simulink model "SailingYachtModelUpdated2"  (R2023b)
settings: Solver=ode3  StartTime=0.0  StopTime=200  FixedStep=0.05  RelTol=1e-3  EnableMultiTasking=on
undefined symbols (not defined in the file or in its folder): par
libraries: simulink_extras x12, vrlib x3
settings Model: Creator=Administrator  LastModifiedBy=henri
settings SolverCC: AlgebraicLoopSolver=TrustRegion
settings DataIOCC: LimitDataPoints=on  SaveFormat=Array  SignalLoggingSaveFormat=ModelDataLogs  ReturnWorkspaceOutputs=off
settings OptimizationCC: ExpressionDepthLimit=2147483647  InitFltsAndDblsToZero=on  LifeSpan=inf
settings DebuggingCC: SaveWithParameterizedLinksMsg=none  UnderspecifiedInitializationDetection=Classic  MergeDetectMultiDrivingBlocksExec=none  SignalResolutionControl=TryResolveAllWithWarning  SolverPrmCheckMsg=warning  MultiTaskDSMMsg=warning  MultiTaskCondExecSysMsg=none  FcnCallInpInsideContextMsg=warning  UnconnectedInputMsg=warning  UnconnectedOutputMsg=warning  UnconnectedLineMsg=warning  StateNameClashWarn=warning  SFUnexpectedBacktrackingDiag=warning  SFNoUnconditionalDefaultTransitionDiag=warning  SFExecutionAtInitializationDiag=none  ArithmeticOperatorsInVariantConditions=warning
settings HardwareCC: ProdBitPerPointer=32  ProdBitPerSizeT=32  ProdBitPerPtrDiffT=32  ProdLargestAtomicFloat=None  ProdIntDivRoundTo=Undefined  ProdEndianess=Unspecified  ProdWordSize=32  ProdHWDeviceType=32-bit Generic
settings ModelReferenceCC: PropagateSignalLabelsOutOfModel=off
settings SFSimCC: SimUseLocalCustomCode=off  CustomCodeUndefinedFunction=UseInterfaceOnly
settings RTWCC: RTWUseLocalCustomCode=off
settings CodeAppCC: StateflowObjectComments=on
settings GRTTargetCC: TargetFcnLib=ansi_tfl_tmw.mat  TargetLangStandard=C89/C90 (ANSI)  CombineOutputUpdateFcns=off  GRTInterface=on
settings ConfigComp: CovMetricSettings=dw  CovSaveCumulativeToWorkspaceVar=on  CovSaveSingleToWorkspaceVar=on  CovExternalEMLEnable=off

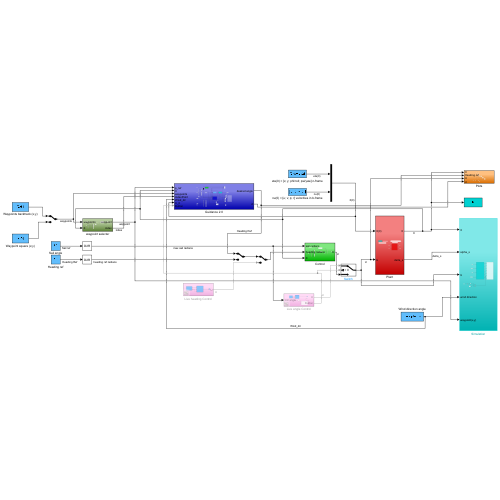
[thumbnail: Simulink's stored preview of the top-level diagram]
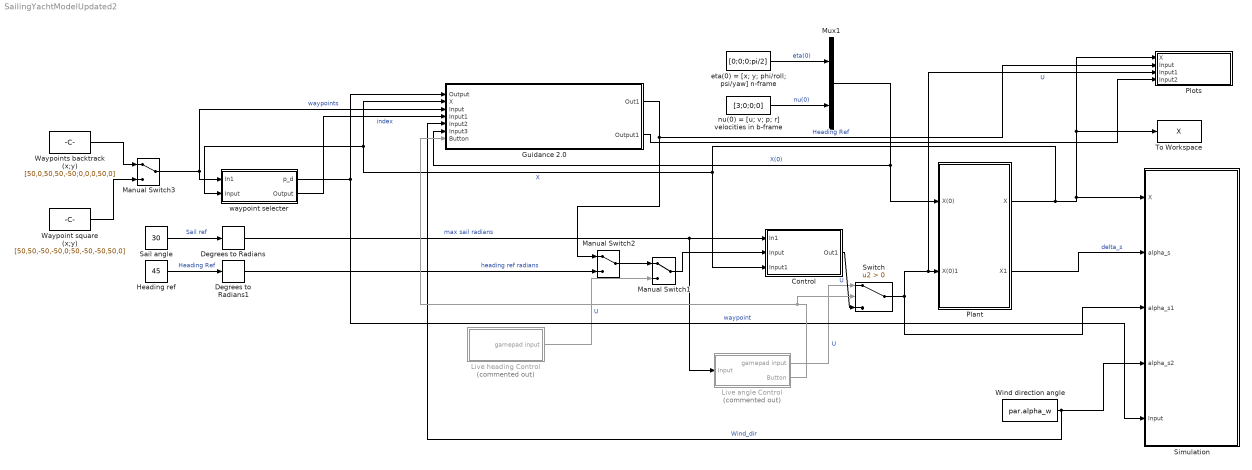
== system SailingYachtModelUpdated2 ==
  Control : Subsystem
  Degrees to Radians : simulink_extras/Transformations/Degrees to Radians
  Degrees to Radians1 : simulink_extras/Transformations/Degrees to Radians
  Guidance 2.0 : Subsystem
  Heading ref : Constant  Value=45
  Live angle Control : Subsystem  Commented=on
  Live heading Control : Subsystem  Commented=on
  Manual Switch1 : ManualSwitch
  Manual Switch2 : ManualSwitch
  Manual Switch3 : ManualSwitch
  Mux1 : Mux  Inputs=2
  Plant : Subsystem
  Plots : Subsystem
  Sail angle : Constant  Value=30
  Simulation : Subsystem
  Switch : Switch  Criteria=u2 > Threshold  SaturateOnIntegerOverflow=off  InputSameDT=off
  To Workspace : ToWorkspace  VariableName=X  SaveFormat=Structure With Time  SampleTime=-1
  Waypoint square (x;y) : Constant  Value=[50,50,-50,-50,0;50,-50,-50,50,0]  VectorParams1D=off
  Waypoints backtrack (x;y) : Constant  Value=[50,0,50,50,-50;0,0,0,50,0]  VectorParams1D=off
  Wind direction angle : Constant  Value=par.alpha_w
  eta(0) = [x; y; phi/roll; psi/yaw] n-frame : Constant  Value=[0;0;0;pi/2]
  nu(0) = [u; v; p; r] velocities in b-frame : Constant  Value=[3;0;0;0]
  waypoint selecter : Subsystem
  wires:
  Mux1/1 -> Plant/1(X(0)), Guidance 2.0/6(Input3)  "X(0)"
  Switch/1 -> Plots/3(Input1), Plant/2(X(0)1), Simulation/3(alpha_s1)  "U"
  Plant/1(X) -> Guidance 2.0/2(X), waypoint selecter/2(Input), Control/3(Input1), Plots/1(X), To Workspace/1, Simulation/1(X)  "X"
  Heading ref/1 -> Degrees to Radians1/1  "Heading Ref"
  Plant/2(X1) -> Simulation/2(alpha_s)  "delta_s"
  Wind direction angle/1 -> Guidance 2.0/5(Input2), Simulation/4(alpha_s2)  "Wind_dir"
  eta(0) = [x; y; phi/roll; psi/yaw] n-frame/1 -> Mux1/1  "eta(0)"
  nu(0) = [u; v; p; r] velocities in b-frame/1 -> Mux1/2  "nu(0)"
  Degrees to Radians/1 -> Live angle Control/1(Input), Control/1(In1)  "max sail radians"
  Sail angle/1 -> Degrees to Radians/1  "Sail ref"
  Degrees to Radians1/1 -> Manual Switch2/2  "heading ref radians"
  Live angle Control/1(gamepad input) -> Switch/1  "U"
  Control/1(Out1) -> Switch/3  "U"
  Live heading Control/1(gamepad input) -> Manual Switch1/2  "U"
  Manual Switch1/1 -> Control/2(Input)
  Manual Switch2/1 -> Manual Switch1/1
  waypoint selecter/1(p_d) -> Simulation/5(Input), Guidance 2.0/1(Output)  "waypoint"
  waypoint selecter/2(Output) -> Guidance 2.0/4(Input1)  "index"
  Guidance 2.0/1(Out1) -> Manual Switch2/1, Plots/2(Input)  "Heading Ref"
  Manual Switch3/1 -> waypoint selecter/1(In1), Guidance 2.0/3(Input)  "waypoints"
  Waypoint square (x;y)/1 -> Manual Switch3/2
  Waypoints backtrack (x;y)/1 -> Manual Switch3/1
  Guidance 2.0/2(Output1) -> Plots/4(Input2)
  Live angle Control/2(Button) -> Switch/2, Guidance 2.0/7(Button)

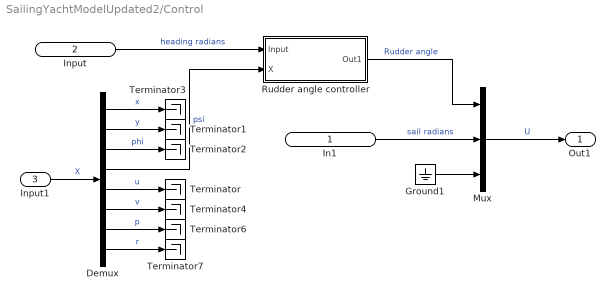
== system SailingYachtModelUpdated2/Control ==
  In1 : Inport
  Input : Inport  Port=2
  Input1 : Inport  Port=3
  Demux : Demux  Outputs=8
  Ground1 : Ground
  Mux : Mux  Inputs=3
  Rudder angle controller : Subsystem
  Terminator{,1..4,6..7} (7 alike) : Terminator
  Out1 : Outport
  wires:
  In1/1 -> Mux/2  "sail radians"
  Rudder angle controller/1(Out1) -> Mux/1  "Rudder angle"
  Mux/1 -> Out1/1  "U"
  Input/1 -> Rudder angle controller/1(Input)  "heading radians"
  Input1/1 -> Demux/1  "X"
  Demux/1 -> Terminator3/1  "x"
  Demux/2 -> Terminator1/1  "y"
  Demux/3 -> Terminator2/1  "phi"
  Demux/4 -> Rudder angle controller/2(X)  "psi"
  Demux/5 -> Terminator/1  "u"
  Demux/6 -> Terminator4/1  "v"
  Demux/7 -> Terminator6/1  "p"
  Demux/8 -> Terminator7/1  "r"
  Ground1/1 -> Mux/3

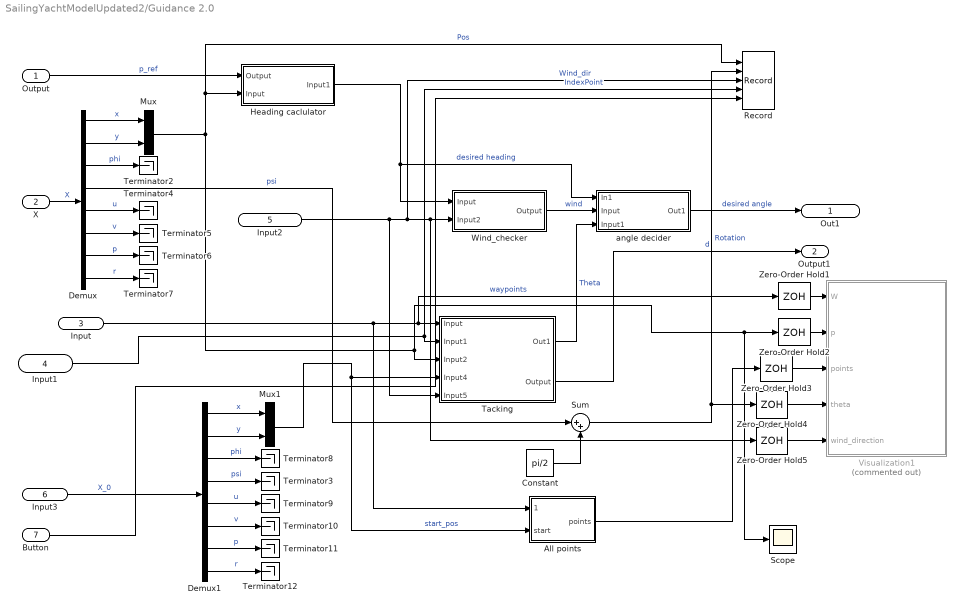
== system SailingYachtModelUpdated2/Guidance 2.0 ==
  Output : Inport
  X : Inport  Port=2
  Input : Inport  Port=3
  Input1 : Inport  Port=4
  Input2 : Inport  Port=5
  Input3 : Inport  Port=6
  Button : Inport  Port=7
  All points : MATLAB Function  TreatAsAtomicUnit=on
  Constant : Constant  Value=pi/2
  Demux : Demux  Outputs=8
  Demux1 : Demux  Outputs=8
  Heading caclulator : Subsystem
  Mux : Mux  Inputs=2
  Mux1 : Mux  Inputs=2
  Record : Record  Filename=C:\Users\henri\OneDrive - Syddansk Universitet\8. Semester\GNC\Assignment_finalV3\AutoRouteFrontBack.xlsx  RecordToFile=on  FileSettingsInternal="{\"entries\":[{\"content\":{\"excelSettings\":{\"content\":{},\"type\":\"Streamout.ExcelSettings\"}},\"type\":\"Streamout.FileSettingStorage\",\"uuid\":\"\"}],\"packageUris\":[\"http:\\/\\/schema.mathworks.com\\/mf0\\/streamout_blocks\\/R2020a\"],\"version\":\"1.0\"}"  SignalsInternal="{\"entries\":[{\"content\":{\"signals\":[{\"content\":{\"blockPath\":[],\"dimensions\":[2],\"domain\":\"\",\"hasChildren\":true,\"lineColor\":\"#ff13a6\",\"port\":1,\"sid\":[\"\"],\"signalID\":899,\"signalName\":\"Pos\"},\"type\":\"RecordBlkView.Signal\",\"uuid\":\"\"},{\"content\":{\"blockPath\":[],\"channel\":[1],\"dimensions\":[2],\"domain\":\"\",\"lineColor\":\"#22b573\",\"parentID\":899,\"plots\":[1],\"port\":1,\"sid\":[\"\"],\"signalID\":900,\"signalName\":\"Pos\"},\"type\":\"RecordBlkView.Signal\",\"uuid\":\"\"},{\"content\":{\"blockPath\":[],\"dimensions\":[1],\"domain\":\"\",\"lineColor\":\"#139fff\",\"plots\":[1],\"port\":2,\"sid\":[\"\"],\"signalID\":904,\"signalName\":\"Rotation\"},\"type\":\"RecordBlkView.Signal\",\"uuid\":\"\"},{\"content\":{\"blockPath\":[],\"dimensions\":[1],\"domain\":\"\",\"lineColor\":\"#b746ff\",\"plots\":[1],\"port\":4,\"sid\":[\"\"],\"signalID\":908,\"signalName\":\"IndexPoint\"},\"type\":\"RecordBlkView.Signal\",\"uuid\":\"\"},{\"content\":{\"blockPath\":[],\"dimensions\":[1],\"domain\":\"\",\"lineColor\":\"#ff6929\",\"plots\":[1],\"port\":3,\"sid\":[\"\"],\"signalID\":912,\"signalName\":\"Wind_dir\"},\"type\":\"RecordBlkView.Signal\",\"uuid\":\"\"},{\"content\":{\"blockPath\":[],\"dimensions\":[1],\"domain\":\"\",\"lineColor\":\"#ff6929\",\"plots\":[1],\"port\":5,\"sid\":[\"\"],\"signalID\":916,\"signalName\":\"Button\"},\"type\":\"RecordBlkView.Signal\",\"uuid\":\"\"},{\"content\":{\"blockPath\":[],\"channel\":[2],\"dimensions\":[2],\"domain\":\"\",\"lineColor\":\"#7e2f8e\",\"parentID\":899,\"plots\":[1],\"port\":1,\"sid\":[\"\"],\"signalID\":921,\"signalName\":\"Pos\"},\"type\":\"RecordBlkView.Signal\",\"uuid\":\"\"}]},\"type\":\"RecordBlkView.InputSignals\",\"uuid\":\"\"}],\"packageUris\":[\"http:\\/\\/schema.mathworks.com\\/mf0\\/streamout_blocks\\/R2020a\"],\"version\":\"1.0\"}"  VisualizationBindings="{\"sparklinesplugin\":{\"info\":[{\"bindingParametersList\":[],\"subplotID\":1}]}}"
  Scope : Scope
  Sum : Sum  Inputs=|++
  Tacking : Subsystem
  Terminator{2..12} (11 alike) : Terminator
  Visualization1 : MATLAB Function  Commented=on  TreatAsAtomicUnit=on
  Wind_checker : Subsystem
  Zero-Order Hold{1..5} (5 alike) : ZeroOrderHold  SampleTime=0.1
  angle decider : Subsystem
  Out1 : Outport
  Output1 : Outport  Port=2
  wires:
  Output/1 -> Heading caclulator/1(Output)  "p_ref"
  Demux/8 -> Terminator7/1  "r"
  Demux/7 -> Terminator6/1  "p"
  Demux/4 -> Sum/1  "psi"
  Demux/3 -> Terminator2/1  "phi"
  Demux/5 -> Terminator4/1  "u"
  X/1 -> Demux/1  "X"
  Demux/2 -> Mux/2  "y"
  Demux/1 -> Mux/1  "x"
  Demux/6 -> Terminator5/1  "v"
  Mux/1 -> Record/1, Heading caclulator/2(Input), Scope/1, Zero-Order Hold2/1, Tacking/3(Input2)  "Pos"
  Input/1 -> All points/1(waypoints), Zero-Order Hold1/1, Tacking/1(Input)  "waypoints"
  Input1/1 -> Record/4, Tacking/2(Input1)  "IndexPoint"
  Heading caclulator/1(Input1) -> angle decider/1(In1), Wind_checker/1(Input)  "desired heading"
  Input2/1 -> Tacking/5(Input5), Record/3, Zero-Order Hold5/1, Wind_checker/2(Input2)  "Wind_dir"
  angle decider/1(Out1) -> Out1/1  "desired angle"
  Wind_checker/1(Output) -> angle decider/2(Input)  "wind"
  Tacking/1(Out1) -> angle decider/3(Input1)  "Theta"
  Input3/1 -> Demux1/1  "X_0"
  Demux1/5 -> Terminator9/1  "u"
  Demux1/3 -> Terminator8/1  "phi"
  Demux1/8 -> Terminator12/1  "r"
  Demux1/7 -> Terminator11/1  "p"
  Demux1/6 -> Terminator10/1  "v"
  Demux1/4 -> Terminator3/1  "psi"
  Demux1/1 -> Mux1/1  "x"
  Demux1/2 -> Mux1/2  "y"
  Mux1/1 -> All points/2(start), Tacking/4(Input4)  "start_pos"
  Constant/1 -> Sum/2
  All points/1(points) -> Zero-Order Hold3/1
  Zero-Order Hold1/1 -> Visualization1/1(W)
  Zero-Order Hold2/1 -> Visualization1/2(p)
  Zero-Order Hold3/1 -> Visualization1/3(points)
  Zero-Order Hold4/1 -> Visualization1/4(theta)
  Zero-Order Hold5/1 -> Visualization1/5(wind_direction)
  Sum/1 -> Zero-Order Hold4/1, Record/2  "Rotation"
  Tacking/2(Output) -> Output1/1  "d"
  Button/1 -> Record/5

== system SailingYachtModelUpdated2/Live angle Control ==
  Input : Inport
  Formatting : Subsystem
  Gamepad : vrlib/Joystick Input  joyid=1  adjustports=on  forcefeed=off
  MATLAB Function : MATLAB Function  TreatAsAtomicUnit=on
  Selector : Selector  InputPortWidth=10  IndexOptions=Index vector (dialog)  Indices=[5]  OutputSizes=1
  gamepad input : Outport
  Button : Outport  Port=2
  wires:
  Gamepad/2 -> Formatting/2(Buttons), Selector/1
  Gamepad/1 -> Formatting/1(Axes)
  Formatting/1(gamepad input) -> gamepad input/1  "U"
  Input/1 -> Formatting/4(Input)  "sail angle"
  ? -> Formatting/3(Point of View)
  Selector/1 -> MATLAB Function/1(input)
  MATLAB Function/1(output) -> Button/1

== system SailingYachtModelUpdated2/Live heading Control ==
  Formatting : Subsystem
  Gamepad : vrlib/Joystick Input  joyid=1  adjustports=on  forcefeed=off
  gamepad input : Outport
  wires:
  Gamepad/2 -> Formatting/2(Buttons)
  Gamepad/1 -> Formatting/1(Axes)
  Formatting/1(gamepad input) -> gamepad input/1  "U"
  ? -> Formatting/3(Point of View)

== system SailingYachtModelUpdated2/Plant ==
  note: Jerome Jouffroy, Jiaxi He and Lin Xiao,
      | University of Southern Denmark, 2014.
  note: (program tested in Matlab r2013a, Simulink 8.1, Simulink 3D Animation 7.0)
  note: Simulation of a 4DOF sailing yacht model
  note: (includes wind speed and direction)
  note: (to look at/change the parameters of the sailing yacht
      | model, right-click on this block, then select
      | "Properties.../Callbacks/InitFcn")
  X(0) : Inport
  X(0)1 : Inport  Port=2
  4DOF nonlinear sailing yacht model : Subsystem
  SubSystem2 : Subsystem  InitFcn=|
      | global par
      | par.m = 25900;                         % (kg),mass of the vehicle
      | par.Ixx = 133690;          
      | par.Izz = 24760;      
      | par.Ixz = 2180;                        % moment of inertia
      | par.a11 = 970;   
      | par.a22 = 17430; 
      | par.a44 = 106500;
      | par.a66 = 101650;
      | par.a24 = -13160;
      | par.a26 = -6190; 
      | par.a46 = 4730;                        % (kg),added mass coef.
      | 
      | par.vt = 10;                           % the norm of wind velocity
      | par.alpha_w = pi;                      % the direction of wind (coming from the north, ie going south)
      | 
      | par.rho_a = 1.2;                       % (kg/m^3), air density
      | par.As = 170;                          % (m^2), sail area
      | par.h0 = 0.0005;                       % (m), roughness height
      | par.h1 = 11.58;                        % (m), reference height
      | par.z_s = -11.58;                      % (m), (x,y,z) is the CoE
      | par.xs = 0;
      | par.ys = 0;
      | par.zs = -11.58;                       % (m), (x,y,z) is the CoE
      | par.Xce = 0.6;                         % (m), distance along the mast to the CoE
      | par.Xm = 0.3;                          % (m), x-coordinate of the mast 
      | 
      | par.rho_w = 1025;                      % (kg/m^3), water density
      | par.Ar = 1.17;                         % (m^2), rudder area
      | par.d_r = 1.9;                         % rudder draft
      | par.zeta_r = 0.8;                      % rudder efficiency
      | par.x_r = -8.2;
      | par.z_r = -0.78;                       % (m), (x,y,z) is the CoE
      | par.xr = -8.2;
      | par.yr = 0;
      | par.zr = -0.78;                        % (m), (x,y,z) is the CoE
      | 
      | par.Ak = 8.7;                          % (m^2), keel area
      | par.d_k = 2.49;                        % keel draft
      | par.zeta_k = 0.7;                      % keel efficiency
      | par.x_k = 0;
      | par.z_k = -0.58;                       % (m), (x,y,z) is the CoE
      | par.xk = 0;
      | par.yk = 0;
      | par.zk = -0.58;                        % (m), (x,y,z) is the CoE
      | 
      | par.x_h = 0;
      | par.z_h = -1.18;                       % (m), (x,y,z) is the CoE
      | par.xh = 0;
      | par.yh = 0;
      | par.zh = -1.18;                        % (m), (x,y,z) is the CoE
      | 
      | par.w_c = 60000;                       % (N), crew weight 20000
      | par.x_c = -8;                          % (m), crew position
      | par.y_bm = 3.6;                        % (m), yacht beam
      | 
      | par.a = -5.89;
      | par.b = 8160;
      | par.c = 120000;
      | par.d = 50000;
      mask Display: disp('Parameter Initialization')
  X : Outport
  X1 : Outport  Port=2
  wires:
  X(0)/1 -> 4DOF nonlinear sailing yacht model/1(X(0))  "X(0)"
  X(0)1/1 -> 4DOF nonlinear sailing yacht model/2(U)  "U"
  4DOF nonlinear sailing yacht model/1(X) -> X/1  "X"
  4DOF nonlinear sailing yacht model/2(delta_s) -> X1/1  "delta_s"

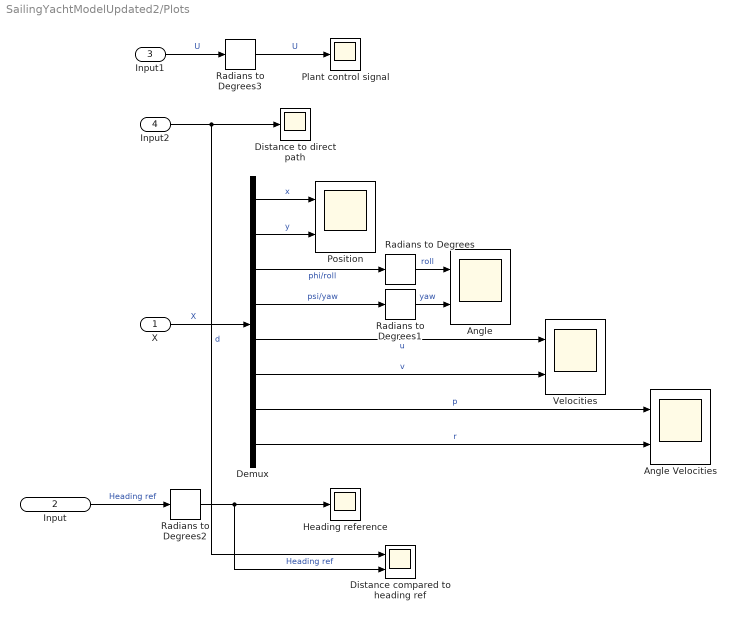
== system SailingYachtModelUpdated2/Plots ==
  X : Inport
  Input : Inport  Port=2
  Input1 : Inport  Port=3
  Input2 : Inport  Port=4
  Angle : Scope  NumInputPorts=2
  Angle Velocities : Scope  NumInputPorts=2
  Demux : Demux  Outputs=8
  Distance compared to heading ref : Scope  NumInputPorts=2
  Distance to direct path : Scope
  Heading reference : Scope
  Plant control signal : Scope
  Position : Scope  NumInputPorts=2
  Radians to Degrees{,1..3} (4 alike) : simulink_extras/Transformations/Radians to Degrees
  Velocities : Scope  NumInputPorts=2
  wires:
  X/1 -> Demux/1  "X"
  Demux/1 -> Position/1  "x"
  Demux/2 -> Position/2  "y"
  Demux/3 -> Radians to Degrees/1  "phi/roll"
  Demux/4 -> Radians to Degrees1/1  "psi/yaw"
  Demux/5 -> Velocities/1  "u"
  Demux/6 -> Velocities/2  "v"
  Demux/7 -> Angle Velocities/1  "p"
  Demux/8 -> Angle Velocities/2  "r"
  Radians to Degrees/1 -> Angle/1  "roll"
  Radians to Degrees1/1 -> Angle/2  "yaw"
  Radians to Degrees2/1 -> Distance compared to heading ref/2, Heading reference/1  "Heading ref"
  Input/1 -> Radians to Degrees2/1  "Heading ref"
  Input1/1 -> Radians to Degrees3/1  "U"
  Radians to Degrees3/1 -> Plant control signal/1  "U"
  Input2/1 -> Distance compared to heading ref/1, Distance to direct path/1  "d"

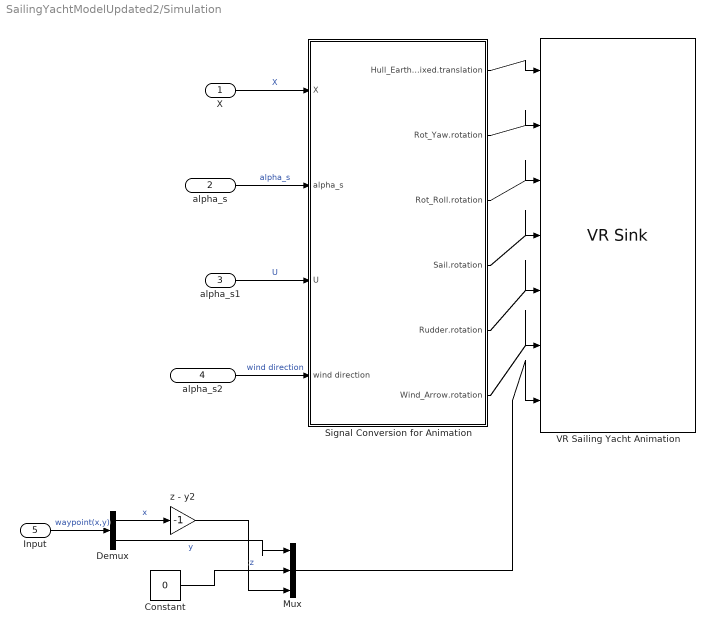
== system SailingYachtModelUpdated2/Simulation ==
  X : Inport
  alpha_s : Inport  Port=2
  alpha_s1 : Inport  Port=3
  alpha_s2 : Inport  Port=4
  Input : Inport  Port=5
  Constant : Constant  Value=0
  Demux : Demux  Outputs=2
  Mux : Mux  Inputs=3
  Signal Conversion for Animation : Subsystem
  VR Sailing Yacht Animation : vrlib/VR Sink  InstantiateOnLoad=on  SampleTime=-1  ViewEnable=on  RemoteChange=off  RemoteView=off  FieldsWritten=Hull_EarthFixed.translation.3.1.1.double#Rot_Yaw.rotation.4.1.1.double#Rot_Roll.rotation.4.1.1.double#Sail.rotation.4.1.1.double#Rudder.rotation.4.1.1.double#Wind_Arrow.rotation.4.1.1.double#Goal.translation.3.1.1.double  WorldFileName=SailingYachtAnimation.wrl  WorldDescription=Sailing Yacht VR animation  AutoView=on  VideoDimensions=[]  AllowVariableSize=off  FigureProperties="{'Position', 'Name', 'Viewpoint', 'CameraBound', 'CameraDirection', 'CameraPosition', 'CameraUpVector', 'ZoomFactor', 'Antialiasing', 'Headlight', 'Lighting', 'NavPanel', 'Sound', 'StatusBar', 'Stereo3D', 'Stereo3DCameraOffset', 'Stereo3DHIT', 'ToolBar', 'Textures', 'Transparency', 'Triad', 'Wireframe', 'NavZones', 'NavMode', 'NavSpeed', 'CaptureFileFormat', 'CaptureFileName', 'Record2DCompressMethod', 'Record2DCompressQuality', 'Record2D', 'Record2DFileName', 'Record2DFPS'; [1.0000000000000000e+00   7.0428571428571331e+01   1.6457142857142856e+03   8.5914285714285711e+02], 'Sailing Yacht VR animation', 'overview', 'on', [-9.2949439619242860e-02  -2.0799088096531138e-01  -9.7370436740816557e-01], [8.2744934194804856e+00   2.5687147459195728e+01   8.2714747859422729e+01], [-9.9855685947730592e-03   9.7808357513325095e-01  -2.0797309555418153e-01], [1.0000000000000000e+00], 'on', 'on', 'on', 'halfbar', 'on', 'on', 'off', [9.0000003576278687e-02], [0.0000000000000000e+00], 'on', 'on', 'on', 'none', 'off', 'off', 'fly', 'normal', 'tif', '%f_anim_%n.tif', 'auto', [7.5000000000000000e+01], 'on', 'AutoRouteFrontBack', [6.0000000000000000e+01]}"
  z - y2 : Gain  Gain=-1
  wires:
  X/1 -> Signal Conversion for Animation/1(X)  "X"
  alpha_s/1 -> Signal Conversion for Animation/2(alpha_s)  "alpha_s"
  alpha_s1/1 -> Signal Conversion for Animation/3(U)  "U"
  alpha_s2/1 -> Signal Conversion for Animation/4(wind direction)  "wind direction"
  Input/1 -> Demux/1  "waypoint(x,y)"
  Constant/1 -> Mux/2  "z"
  Demux/1 -> z - y2/1  "x"
  Demux/2 -> Mux/1  "y"
  z - y2/1 -> Mux/3
  Signal Conversion for Animation/1(Hull_EarthFixed.translation) -> VR Sailing Yacht Animation/1
  Signal Conversion for Animation/2(Rot_Yaw.rotation) -> VR Sailing Yacht Animation/2
  Signal Conversion for Animation/3(Rot_Roll.rotation) -> VR Sailing Yacht Animation/3
  Signal Conversion for Animation/4(Sail.rotation) -> VR Sailing Yacht Animation/4
  Signal Conversion for Animation/5(Rudder.rotation) -> VR Sailing Yacht Animation/5
  Signal Conversion for Animation/6(Wind_Arrow.rotation) -> VR Sailing Yacht Animation/6
  Mux/1 -> VR Sailing Yacht Animation/7

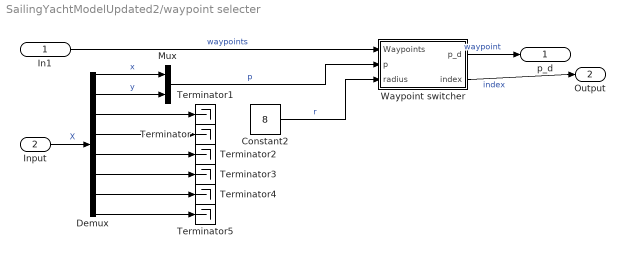
== system SailingYachtModelUpdated2/waypoint selecter ==
  In1 : Inport
  Input : Inport  Port=2
  Constant2 : Constant  Value=8
  Demux : Demux  Outputs=8
  Mux : Mux  Inputs=2
  Terminator{,1..5} (6 alike) : Terminator
  Waypoint switcher : MATLAB Function  TreatAsAtomicUnit=on
  p_d : Outport
  Output : Outport  Port=2
  wires:
  Constant2/1 -> Waypoint switcher/3(radius)  "r"
  In1/1 -> Waypoint switcher/1(Waypoints)  "waypoints"
  Mux/1 -> Waypoint switcher/2(p)  "p"
  Waypoint switcher/1(p_d) -> p_d/1  "waypoint"
  Input/1 -> Demux/1  "X"
  Demux/1 -> Mux/1  "x"
  Demux/2 -> Mux/2  "y"
  Demux/4 -> Terminator/1
  Demux/3 -> Terminator1/1
  Demux/5 -> Terminator2/1
  Demux/6 -> Terminator3/1
  Demux/7 -> Terminator4/1
  Demux/8 -> Terminator5/1
  Waypoint switcher/2(index) -> Output/1  "index"

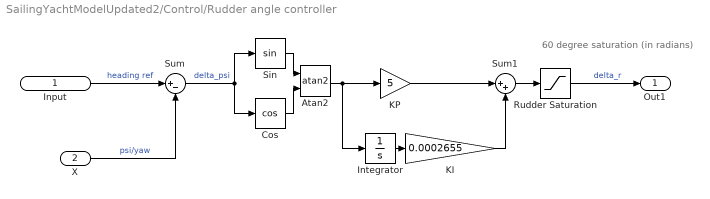
== system SailingYachtModelUpdated2/Control/Rudder angle controller ==
  note: 60 degree saturation (in radians)
  Input : Inport
  X : Inport  Port=2
  Atan2 : Trigonometry  Operator=atan2
  Cos : Trigonometry  Operator=cos
  Integrator : Integrator
  KI : Gain  Gain=0.0002655
  KP : Gain  Gain=5
  Rudder Saturation : Saturate  UpperLimit=pi/3  LowerLimit=-pi/3
  Sin : Trigonometry
  Sum : Sum  Inputs=|+-
  Sum1 : Sum  Inputs=|++
  Out1 : Outport
  wires:
  Input/1 -> Sum/1  "heading ref"
  X/1 -> Sum/2  "psi/yaw"
  Sum/1 -> Cos/1, Sin/1  "delta_psi"
  KP/1 -> Sum1/1
  Rudder Saturation/1 -> Out1/1  "delta_r"
  Sum1/1 -> Rudder Saturation/1
  KI/1 -> Sum1/2
  Integrator/1 -> KI/1
  Atan2/1 -> Integrator/1, KP/1
  Sin/1 -> Atan2/1
  Cos/1 -> Atan2/2

== system SailingYachtModelUpdated2/Guidance 2.0/Heading caclulator ==
  Output : Inport
  Input : Inport  Port=2
  Atan2 : Trigonometry  Operator=atan2
  Demux : Demux  Outputs=2
  Sum : Sum  Inputs=|+-
  Input1 : Outport
  wires:
  Output/1 -> Sum/1  "p_ref"
  Input/1 -> Sum/2  "p"
  Demux/1 -> Atan2/2  "delta_x"
  Demux/2 -> Atan2/1  "delta_y"
  Sum/1 -> Demux/1  "delta_p"
  Atan2/1 -> Input1/1  "desired"

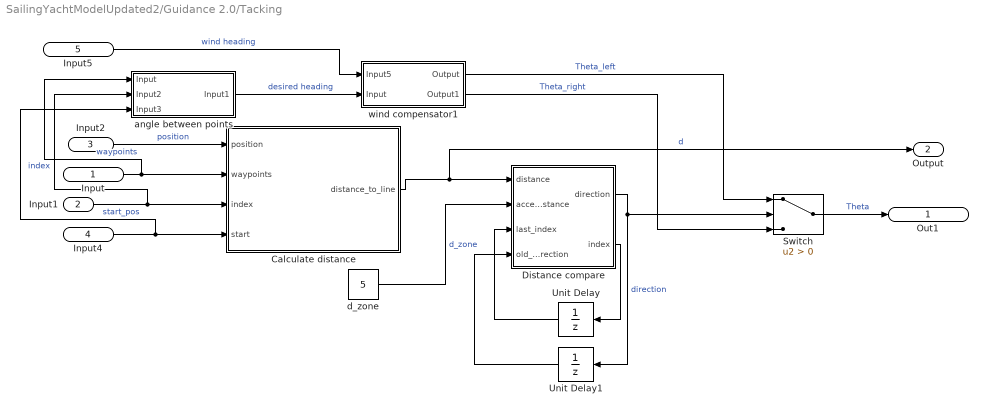
== system SailingYachtModelUpdated2/Guidance 2.0/Tacking ==
  Input : Inport
  Input1 : Inport  Port=2
  Input2 : Inport  Port=3
  Input4 : Inport  Port=4
  Input5 : Inport  Port=5
  Calculate distance : MATLAB Function  TreatAsAtomicUnit=on
  Distance compare : MATLAB Function  TreatAsAtomicUnit=on
  Switch : Switch  Criteria=u2 > Threshold  SaturateOnIntegerOverflow=off  InputSameDT=off
  Unit Delay : UnitDelay  SampleTime=-1  HasFrameUpgradeWarning=on
  Unit Delay1 : UnitDelay  InitialCondition=1  SampleTime=-1  HasFrameUpgradeWarning=on
  angle between points : Subsystem
  d_zone : Constant  Value=5
  wind compensator1 : Subsystem
  Out1 : Outport
  Output : Outport  Port=2
  wires:
  Input/1 -> angle between points/1(Input), Calculate distance/2(waypoints)  "waypoints"
  Input1/1 -> angle between points/2(Input2), Calculate distance/3(index)  "index"
  Input2/1 -> Calculate distance/1(position)  "position"
  Calculate distance/1(distance_to_line) -> Output/1, Distance compare/1(distance)  "d"
  d_zone/1 -> Distance compare/2(acceptzone_distance)  "d_zone"
  Distance compare/1(direction) -> Unit Delay1/1, Switch/2  "direction"
  Input4/1 -> angle between points/3(Input3), Calculate distance/4(start)  "start_pos"
  Unit Delay/1 -> Distance compare/3(last_index)
  Distance compare/2(index) -> Unit Delay/1
  Unit Delay1/1 -> Distance compare/4(old_direction)
  Switch/1 -> Out1/1  "Theta"
  Input5/1 -> wind compensator1/1(Input5)  "wind heading"
  angle between points/1(Input1) -> wind compensator1/2(Input)  "desired heading"
  wind compensator1/1(Output) -> Switch/1  "Theta_left"
  wind compensator1/2(Output1) -> Switch/3  "Theta_right"

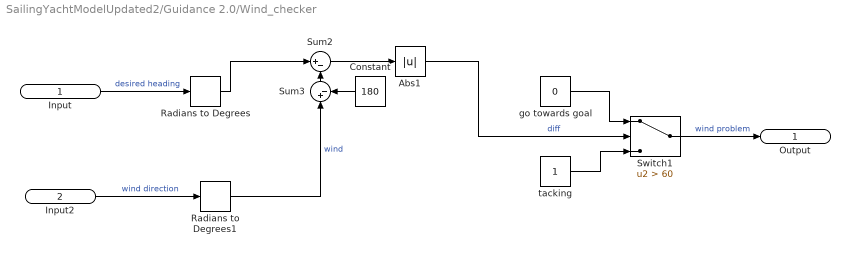
== system SailingYachtModelUpdated2/Guidance 2.0/Wind_checker ==
  Input : Inport
  Input2 : Inport  Port=2
  Abs1 : Abs  SaturateOnIntegerOverflow=off
  Constant : Constant  Value=180
  Radians to Degrees : simulink_extras/Transformations/Radians to Degrees
  Radians to Degrees1 : simulink_extras/Transformations/Radians to Degrees
  Sum2 : Sum  Inputs=|+-
  Sum3 : Sum  Inputs=|+-
  Switch1 : Switch  Criteria=u2 > Threshold  Threshold=60  SaturateOnIntegerOverflow=off  InputSameDT=off
  go towards goal : Constant  Value=0
  tacking : Constant
  Output : Outport
  wires:
  Sum3/1 -> Sum2/2
  tacking/1 -> Switch1/3
  Sum2/1 -> Abs1/1
  Abs1/1 -> Switch1/2  "diff"
  go towards goal/1 -> Switch1/1
  Constant/1 -> Sum3/2
  Radians to Degrees1/1 -> Sum3/1  "wind"
  Switch1/1 -> Output/1  "wind problem"
  Radians to Degrees/1 -> Sum2/1
  Input2/1 -> Radians to Degrees1/1  "wind direction"
  Input/1 -> Radians to Degrees/1  "desired heading"

== system SailingYachtModelUpdated2/Guidance 2.0/angle decider ==
  In1 : Inport
  Input : Inport  Port=2
  Input1 : Inport  Port=3
  Switch : Switch  Criteria=u2 > Threshold  SaturateOnIntegerOverflow=off  InputSameDT=off
  Out1 : Outport
  wires:
  Input1/1 -> Switch/1  "Theta"
  Input/1 -> Switch/2  "wind"
  In1/1 -> Switch/3  "desired"
  Switch/1 -> Out1/1  "Desired angle"

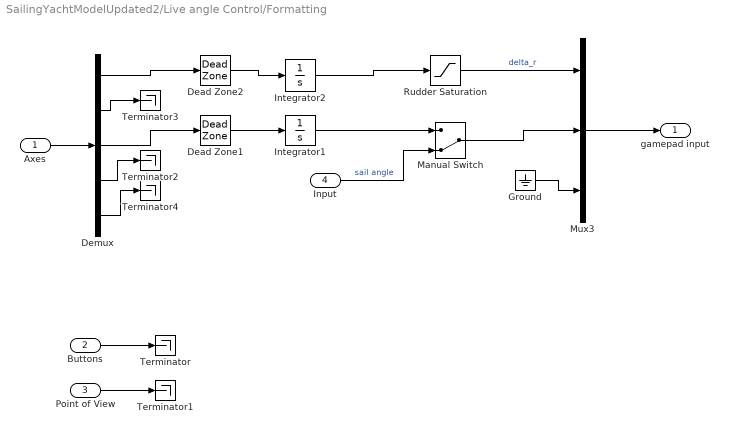
== system SailingYachtModelUpdated2/Live angle Control/Formatting ==
  Axes : Inport
  Buttons : Inport  Port=2
  Point of View : Inport  Port=3
  Input : Inport  Port=4
  Dead Zone1 : DeadZone  LowerValue=-0.2  UpperValue=0.2
  Dead Zone2 : DeadZone  LowerValue=-0.2  UpperValue=0.2
  Demux : Demux  Outputs=5
  Ground : Ground
  Integrator1 : Integrator
  Integrator2 : Integrator
  Manual Switch : ManualSwitch  CurrentSetting=0
  Mux3 : Mux  Inputs=3
  Rudder Saturation : Saturate  UpperLimit=pi/3  LowerLimit=-pi/3
  Terminator{,1..4} (5 alike) : Terminator
  gamepad input : Outport
  wires:
  Mux3/1 -> gamepad input/1
  Buttons/1 -> Terminator/1
  Axes/1 -> Demux/1
  Demux/3 -> Dead Zone1/1
  Demux/5 -> Terminator4/1
  Demux/4 -> Terminator2/1
  Point of View/1 -> Terminator1/1
  Demux/1 -> Dead Zone2/1
  Ground/1 -> Mux3/3
  Demux/2 -> Terminator3/1
  Integrator2/1 -> Rudder Saturation/1
  Dead Zone2/1 -> Integrator2/1
  Dead Zone1/1 -> Integrator1/1
  Rudder Saturation/1 -> Mux3/1  "delta_r"
  Integrator1/1 -> Manual Switch/1
  Manual Switch/1 -> Mux3/2
  Input/1 -> Manual Switch/2  "sail angle"

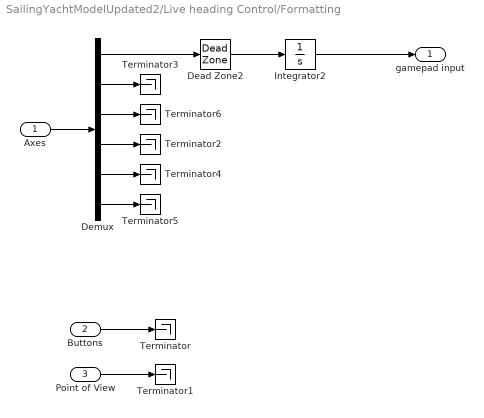
== system SailingYachtModelUpdated2/Live heading Control/Formatting ==
  Axes : Inport
  Buttons : Inport  Port=2
  Point of View : Inport  Port=3
  Dead Zone2 : DeadZone  LowerValue=-0.2  UpperValue=0.2
  Demux : Demux  Outputs=6
  Integrator2 : Integrator  InitialCondition=pi/2
  Terminator{,1..6} (7 alike) : Terminator
  gamepad input : Outport
  wires:
  Integrator2/1 -> gamepad input/1
  Buttons/1 -> Terminator/1
  Axes/1 -> Demux/1
  Demux/3 -> Terminator6/1
  Demux/5 -> Terminator4/1
  Demux/6 -> Terminator5/1
  Demux/4 -> Terminator2/1
  Point of View/1 -> Terminator1/1
  Demux/1 -> Dead Zone2/1
  Demux/2 -> Terminator3/1
  Dead Zone2/1 -> Integrator2/1

== system SailingYachtModelUpdated2/Plant/4DOF nonlinear sailing yacht model ==
  note: X_dot
  note: V_in = [U,X]
  X(0) : Inport
  U : Inport  Port=2
  Demux : Demux  Outputs=9
  Integrator : Integrator  InitialConditionSource=external  InitialCondition=[0;0;0;pi;1;0;0;0]
  Mux : Mux  Inputs=2
  Mux1 : Mux  Inputs=8
  X_dot_ext=f(V_in) : MATLABFcn  MATLABFcn=f  OutputDimensions=9
  X : Outport
  delta_s : Outport  Port=2
  wires:
  X(0)/1 -> Integrator/2
  Mux/1 -> X_dot_ext=f(V_in)/1
  U/1 -> Mux/1
  Integrator/1 -> X/1, Mux/2
  X_dot_ext=f(V_in)/1 -> Demux/1
  Demux/9 -> delta_s/1
  Demux/8 -> Mux1/8
  Demux/7 -> Mux1/7
  Demux/6 -> Mux1/6
  Demux/5 -> Mux1/5
  Demux/4 -> Mux1/4
  Demux/3 -> Mux1/3
  Demux/2 -> Mux1/2
  Demux/1 -> Mux1/1
  Mux1/1 -> Integrator/1

== system SailingYachtModelUpdated2/Plant/SubSystem2 ==

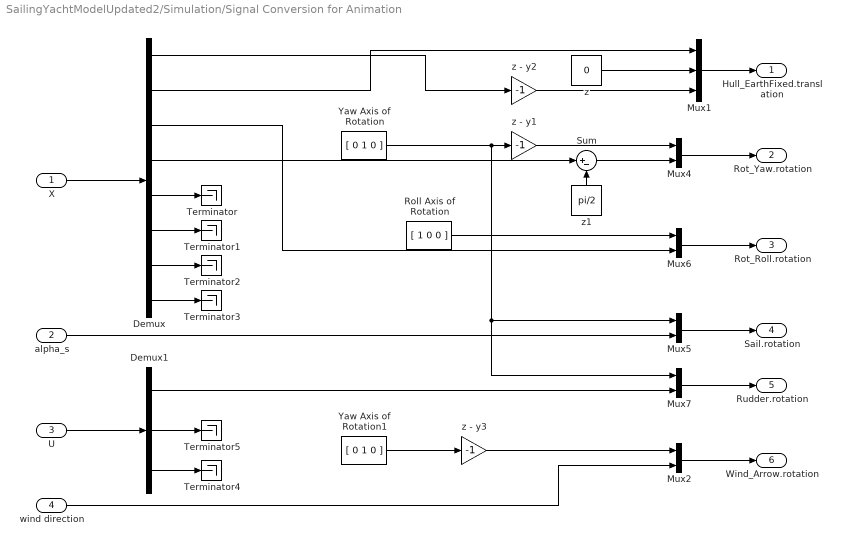
== system SailingYachtModelUpdated2/Simulation/Signal Conversion for Animation ==
  X : Inport
  alpha_s : Inport  Port=2
  U : Inport  Port=3
  wind direction : Inport  Port=4
  Demux : Demux  Outputs=8
  Demux1 : Demux  Outputs=3
  Mux1 : Mux  Inputs=3
  Mux{2,4..7} (5 alike) : Mux  Inputs=2
  Roll Axis of Rotation : Constant  Value=[ 1 0 0 ]
  Sum : Sum  Inputs=|+-  SaturateOnIntegerOverflow=on
  Terminator{,1..5} (6 alike) : Terminator
  Yaw Axis of Rotation : Constant  Value=[ 0 1 0 ]
  Yaw Axis of Rotation1 : Constant  Value=[ 0 1 0 ]
  z : Constant  Value=0
  z - y1 : Gain  Gain=-1
  z - y2 : Gain  Gain=-1
  z - y3 : Gain  Gain=-1
  z1 : Constant  Value=pi/2
  Hull_EarthFixed.translation : Outport
  Rot_Yaw.rotation : Outport  Port=2
  Rot_Roll.rotation : Outport  Port=3
  Sail.rotation : Outport  Port=4
  Rudder.rotation : Outport  Port=5
  Wind_Arrow.rotation : Outport  Port=6
  wires:
  Demux/4 -> Sum/1
  Yaw Axis of Rotation/1 -> Mux5/1, Mux7/1, z - y1/1
  Sum/1 -> Mux4/2
  Roll Axis of Rotation/1 -> Mux6/1
  Demux/3 -> Mux6/2
  alpha_s/1 -> Mux5/2
  Demux/1 -> z - y2/1
  z - y2/1 -> Mux1/3
  Demux/2 -> Mux1/1
  z/1 -> Mux1/2
  z - y1/1 -> Mux4/1
  z1/1 -> Sum/2
  Mux1/1 -> Hull_EarthFixed.translation/1
  Demux/5 -> Terminator/1
  Demux/6 -> Terminator1/1
  Demux/7 -> Terminator2/1
  Demux/8 -> Terminator3/1
  X/1 -> Demux/1
  Demux1/3 -> Terminator4/1
  Demux1/2 -> Terminator5/1
  U/1 -> Demux1/1
  Demux1/1 -> Mux7/2
  Mux7/1 -> Rudder.rotation/1
  Mux5/1 -> Sail.rotation/1
  Mux4/1 -> Rot_Yaw.rotation/1
  Yaw Axis of Rotation1/1 -> z - y3/1
  z - y3/1 -> Mux2/1
  wind direction/1 -> Mux2/2
  Mux2/1 -> Wind_Arrow.rotation/1
  Mux6/1 -> Rot_Roll.rotation/1

== system SailingYachtModelUpdated2/Guidance 2.0/Tacking/angle between points ==
  Input : Inport
  Input2 : Inport  Port=2
  Input3 : Inport  Port=3
  Atan2 : Trigonometry  Operator=atan2
  Demux : Demux  Outputs=2
  MATLAB Function : MATLAB Function  TreatAsAtomicUnit=on
  Sum : Sum  Inputs=|+-
  Input1 : Outport
  wires:
  Demux/1 -> Atan2/2  "delta_x"
  Demux/2 -> Atan2/1  "delta_y"
  Atan2/1 -> Input1/1  "desired"
  Input/1 -> MATLAB Function/1(waypoints)  "waypoints"
  Input2/1 -> MATLAB Function/2(index)  "index"
  Input3/1 -> MATLAB Function/3(start)  "start"
  MATLAB Function/1(point_ref) -> Sum/1
  MATLAB Function/2(point) -> Sum/2
  Sum/1 -> Demux/1

== system SailingYachtModelUpdated2/Guidance 2.0/Tacking/wind compensator1 ==
  Input5 : Inport
  Input : Inport  Port=2
  Constant : Constant  Value=60
  Degrees to Radians : simulink_extras/Transformations/Degrees to Radians
  Degrees to Radians1 : simulink_extras/Transformations/Degrees to Radians
  MATLAB Function : MATLAB Function  TreatAsAtomicUnit=on
  Radians to Degrees : simulink_extras/Transformations/Radians to Degrees
  Radians to Degrees1 : simulink_extras/Transformations/Radians to Degrees
  Output : Outport
  Output1 : Outport  Port=2
  wires:
  Input5/1 -> Radians to Degrees1/1  "wind"
  Input/1 -> Radians to Degrees/1  "heading"
  Radians to Degrees/1 -> MATLAB Function/2(heading)  "heading"
  Constant/1 -> MATLAB Function/1(tacking_angle)  "tacking angle"
  Radians to Degrees1/1 -> MATLAB Function/3(wind_angle)  "wind"
  Degrees to Radians/1 -> Output/1  "heading_left"
  Degrees to Radians1/1 -> Output1/1  "heading_right"
  MATLAB Function/2(tacking_right) -> Degrees to Radians1/1
  MATLAB Function/1(tacking_left) -> Degrees to Radians/1

== matlab function SailingYachtModelUpdated2/waypoint selecter/Waypoint switcher ==
  settings: updateMethod=DISCRETE
  data: Waypoints input; p_d output; p input; radius input; index output
function [p_d,index] = fcn(Waypoints,p,radius)

persistent i;

if isempty(i)
    i = 1;
end

if norm(p-Waypoints(:,i)) < radius && size(Waypoints,2) > i
    i = i+1;
end
index = i;
p_d = Waypoints(:,i);

== matlab function SailingYachtModelUpdated2/Guidance 2.0/All points ==
  data: waypoints input; points output; start input
function points = fcn(waypoints,start)
points = [[start(1);start(2)],waypoints];

== matlab function SailingYachtModelUpdated2/Guidance 2.0/Tacking/wind compensator1/MATLAB Function ==
  data: tacking_angle input; tacking_left output; heading input; wind_angle input; tacking_right output
function [tacking_left,tacking_right] = fcn(tacking_angle,heading,wind_angle)

angle_left = heading+tacking_angle;
angle_right = heading-tacking_angle;

head_wind = wind_angle - 180;

left_diff = max(abs(angle_left-head_wind),abs(head_wind-angle_left));
right_diff = max(abs(angle_right-head_wind),abs(head_wind-angle_right));

if left_diff < tacking_angle
    angle_left = angle_left + tacking_angle-left_diff;
end
if right_diff < tacking_angle
    angle_right = angle_right - tacking_angle+right_diff;
end
tacking_left = angle_left;
tacking_right = angle_right;

== matlab function SailingYachtModelUpdated2/Live angle Control/MATLAB Function ==
  data: input input; output output
function output = toggleOnRisingEdge(input)
persistent prevInput;
persistent prevOutput;

if isempty(prevInput) || isempty(prevOutput)
    % Initialize persistent variables
    prevInput = false;  % Assuming input is logical
    prevOutput = false; % Assuming output is logical
end

% Check for rising edge
if input && ~prevInput
    % Toggle the output
    output = ~prevOutput;
else
    % Output remains unchanged
    output = prevOutput;
end

% Update previous input and output for the next iteration
prevInput = input;
prevOutput = output;
end

== matlab function SailingYachtModelUpdated2/Guidance 2.0/Tacking/Calculate distance ==
  data: position input; distance_to_line output; waypoints input; index input; start input
function distance_to_line = fcn(position,waypoints,index,start)
% Get next point
next_point = waypoints(:,index);
next_x = next_point(1,1);
next_y = next_point(2,1);

% Get last point as start point
last_x = start(1);
last_y = start(2);

% if index is bigger than 1 take last point instead
if index > 1
    last_point = waypoints(:,index-1);
    last_x = last_point(1,1);
    last_y = last_point(2,1);
end

% calculate line to goal
a = (next_y-last_y)/(next_x-last_x);
b = last_y-a*last_x;

% standard form
A = next_y - last_y;
B = last_x - next_x;
C = last_y*(next_x-last_x)-(next_y-last_y)*last_x;

% Get position
x = position(1);
y = position(2);

% calculate sign of line
%distance_sign = sign((next_x-last_x)*(y-last_y)-(next_y-last_y)*(x-last_x)); 

% calculate distance to line
distance_to_line = abs(A*x+B*y+C)/(sqrt(A^2+B^2));

== matlab function SailingYachtModelUpdated2/Guidance 2.0/Tacking/Distance compare ==
  settings: updateMethod=DISCRETE
  data: distance input; direction output; acceptzone_distance input; last_index input; index output; old_direction input
function [direction,index] = fcn(distance,acceptzone_distance,last_index, old_direction)

if distance >= acceptzone_distance
    i = 1;
else
    i = 0;
end

direction = old_direction;

if last_index == 0
    if i == 1
        if old_direction == 1
            direction = 0;
        else
            direction = 1;
        end
    end
end    
index = i;

== matlab function SailingYachtModelUpdated2/Guidance 2.0/Tacking/angle between points/MATLAB Function ==
  data: waypoints input; point_ref output; index input; start input; point output
function [point_ref,point] = fcn(waypoints,index,start)
index_point = waypoints(:,index);
next_x = index_point(1,1);
next_y = index_point(2,1);
last_x = start(1);
last_y = start(2);
if index > 1
    last_point = waypoints(:,index-1);
    last_x = last_point(1,1);
    last_y = last_point(2,1);

end
point_ref = [next_x,next_y];
point = [last_x,last_y];

== matlab function SailingYachtModelUpdated2/Guidance 2.0/Visualization1 ==
  settings: updateMethod=DISCRETE
  data: W input; p input; points input; theta input; wind_direction input
function fcn(W, p, points, theta, wind_direction)

persistent tracer_path_history

x = p(1);
y = p(2);

% Scaling factor for the boat size
scale_factor = 10;

% Body "shape"
Ybody = scale_factor * [-0.4; -0.4; 0.4; 0.4];
Xbody = scale_factor * [-0.2; 0.2; 0.2; -0.2];

% Rotation matrix
R = [cos(theta), -sin(theta); sin(theta), cos(theta)];

% Rotate body vertices
Body = [Xbody'; Ybody'];
Body = R * Body;

% Translated and rotated body vertices
PosXbody = Body(1, :) + x;
PosYbody = Body(2, :) + y;

% Plot path
plot(points(1,:),points(2,:));
hold on;
% Plot waypoints
plot(W(1, :), W(2, :), 'o', ...
    'LineWidth', 2, ...
    'MarkerSize', 20, ...
    'MarkerEdgeColor', 'g', ...
    'MarkerFaceColor', [0, 1, 0])

% Draw body of vehicle and axles
fill(PosXbody, PosYbody, 'b');

% Update tracer path
if isempty(tracer_path_history)
    tracer_path_history = p;
else
    tracer_path_history = [tracer_path_history, p];
end

% Plot tracer path (in red)
if size(tracer_path_history, 2) > 1
    plot(tracer_path_history(1, :), tracer_path_history(2, :), 'r--', 'LineWidth', 1);
end


% Draw wind direction arrow
wind_arrow_length = 5;
arrow_dx = wind_arrow_length * cosd(wind_direction + 180);
arrow_dy = wind_arrow_length * sind(wind_direction + 180);
quiver(x-6, y, arrow_dx, arrow_dy, 0, 'black', 'LineWidth', 2, 'MaxHeadSize', 6);


hold off
axis([-60 60 -60 60]);
title('Waypoints, paths, and trajectories');
grid on;
drawnow;
